simulink model "BMS_System"  (R2024a)
settings: Solver=VariableStepAuto  StartTime=0.0  StopTime=10.0  RelTol=1e-3
settings Model: DataDictionary=BMS_System_dict1.sldd  Creator=hirah  LastModifiedBy=hirah

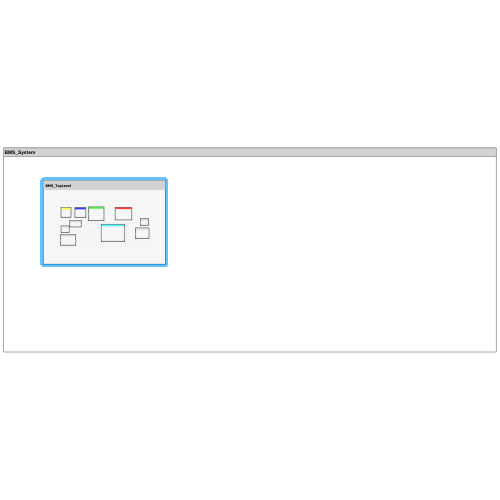
[thumbnail: Simulink's stored preview of the top-level diagram]
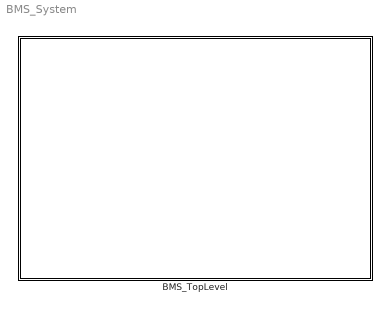
== system BMS_System ==
  BMS_TopLevel : Subsystem
      settings: PortSchema="{\"entries\":[{\"content\":{\"headerSize\":26,\"margin\":15,\"minimumSpacing\":25,\"sides\":[{\"content\":{},\"type\":\"ConnectorPlacement.EquallySpacedRectSide\",\"uuid\":\"0075fff4-e359-4ca3-82d3-62066e5371b3\"},{\"content\":{\"side\":\"RIGHT\"},\"type\":\"ConnectorPlacement.EquallySpacedRectSide\",\"uuid\":\"0762518f-8ff4-47a0-8585-614cecfccf10\"},{\"content\":{\"side\":\"TOP\"},\"type\":\"ConnectorPlacement.EquallySpacedRectSide\",\"uuid\":\"3af96ac8-a5e6-433b-be31-5dc09c2330cd\"}]},\"type\":\"ConnectorPlacement.EquallySpacedConnector\",\"uuid\":\"5c35ae06-51a0-47e4-81f3-25c096dd406a\"}],\"packageUris\":[\"http://schema.mathworks.com/mf0/Connector/R2020b\"],\"version\":\"1.0\"}"

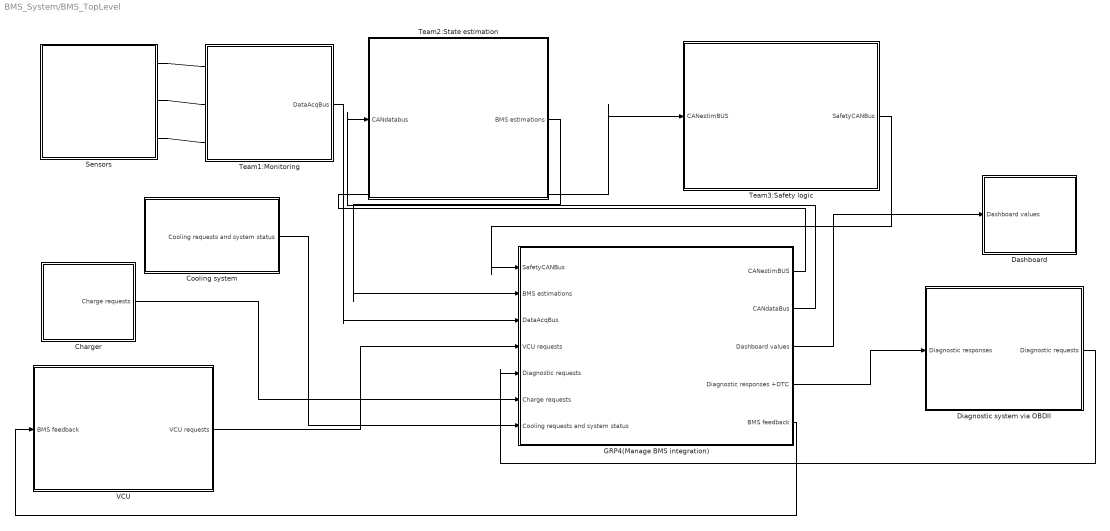
== system BMS_System/BMS_TopLevel ==
  Charger : Subsystem
      settings: PortSchema="{\"entries\":[{\"content\":{\"headerSize\":26,\"margin\":15,\"minimumSpacing\":25,\"sides\":[{\"content\":{},\"type\":\"ConnectorPlacement.EquallySpacedRectSide\",\"uuid\":\"cd2cdd02-8687-4a8c-9b6e-8ab5b03022cf\"},{\"content\":{\"connectorIds\":[\"Out1\"],\"side\":\"RIGHT\"},\"type\":\"ConnectorPlacement.EquallySpacedRectSide\",\"uuid\":\"c7d3337e-acaa-4958-9ee3-86e02c1b3b1e\"},{\"content\":{\"side\":\"TOP\"},\"type\":\"ConnectorPlacement.EquallySpacedRectSide\",\"uuid\":\"181ed1e6-99e4-4d5e-88b9-0d6c177ff349\"}]},\"type\":\"ConnectorPlacement.EquallySpacedConnector\",\"uuid\":\"35383a89-4be3-49fe-8681-3a2efe2b709c\"}],\"packageUris\":[\"http://schema.mathworks.com/mf0/Connector/R2020b\"],\"version\":\"1.0\"}"
  Cooling system : Subsystem
      settings: PortSchema="{\"entries\":[{\"content\":{\"headerSize\":26,\"margin\":15,\"minimumSpacing\":25,\"sides\":[{\"content\":{},\"type\":\"ConnectorPlacement.EquallySpacedRectSide\",\"uuid\":\"cd2cdd02-8687-4a8c-9b6e-8ab5b03022cf\"},{\"content\":{\"connectorIds\":[\"Out1\"],\"side\":\"RIGHT\"},\"type\":\"ConnectorPlacement.EquallySpacedRectSide\",\"uuid\":\"c7d3337e-acaa-4958-9ee3-86e02c1b3b1e\"},{\"content\":{\"side\":\"TOP\"},\"type\":\"ConnectorPlacement.EquallySpacedRectSide\",\"uuid\":\"181ed1e6-99e4-4d5e-88b9-0d6c177ff349\"}]},\"type\":\"ConnectorPlacement.EquallySpacedConnector\",\"uuid\":\"35383a89-4be3-49fe-8681-3a2efe2b709c\"}],\"packageUris\":[\"http://schema.mathworks.com/mf0/Connector/R2020b\"],\"version\":\"1.0\"}"
  Dashboard : Subsystem
      settings: PortSchema="{\"entries\":[{\"content\":{\"headerSize\":26,\"margin\":15,\"minimumSpacing\":25,\"sides\":[{\"content\":{\"connectorIds\":[\"In1\"]},\"type\":\"ConnectorPlacement.EquallySpacedRectSide\",\"uuid\":\"cd2cdd02-8687-4a8c-9b6e-8ab5b03022cf\"},{\"content\":{\"side\":\"RIGHT\"},\"type\":\"ConnectorPlacement.EquallySpacedRectSide\",\"uuid\":\"c7d3337e-acaa-4958-9ee3-86e02c1b3b1e\"},{\"content\":{\"side\":\"TOP\"},\"type\":\"ConnectorPlacement.EquallySpacedRectSide\",\"uuid\":\"181ed1e6-99e4-4d5e-88b9-0d6c177ff349\"}]},\"type\":\"ConnectorPlacement.EquallySpacedConnector\",\"uuid\":\"35383a89-4be3-49fe-8681-3a2efe2b709c\"}],\"packageUris\":[\"http://schema.mathworks.com/mf0/Connector/R2020b\"],\"version\":\"1.0\"}"
  Diagnostic system via OBDII : Subsystem
      settings: PortSchema="{\"entries\":[{\"content\":{\"headerSize\":26,\"margin\":15,\"minimumSpacing\":25,\"sides\":[{\"content\":{\"connectorIds\":[\"In1\"]},\"type\":\"ConnectorPlacement.EquallySpacedRectSide\",\"uuid\":\"cd2cdd02-8687-4a8c-9b6e-8ab5b03022cf\"},{\"content\":{\"connectorIds\":[\"Out1\"],\"side\":\"RIGHT\"},\"type\":\"ConnectorPlacement.EquallySpacedRectSide\",\"uuid\":\"c7d3337e-acaa-4958-9ee3-86e02c1b3b1e\"},{\"content\":{\"side\":\"TOP\"},\"type\":\"ConnectorPlacement.EquallySpacedRectSide\",\"uuid\":\"181ed1e6-99e4-4d5e-88b9-0d6c177ff349\"}]},\"type\":\"ConnectorPlacement.EquallySpacedConnector\",\"uuid\":\"35383a89-4be3-49fe-8681-3a2efe2b709c\"}],\"packageUris\":[\"http://schema.mathworks.com/mf0/Connector/R2020b\"],\"version\":\"1.0\"}"
  GRP4(Manage BMS integration) : Subsystem
      settings: PortSchema="{\"entries\":[{\"content\":{\"headerSize\":26,\"margin\":15,\"minimumSpacing\":25,\"sides\":[{\"content\":{\"connectorIds\":[\"In1\",\"In6\",\"In2\",\"In7\",\"In3\",\"In4\",\"In5\"]},\"type\":\"ConnectorPlacement.EquallySpacedRectSide\",\"uuid\":\"faff89d9-e9e4-4b6f-9f42-f9315910e0de\"},{\"content\":{\"connectorIds\":[\"Out1\",\"Out2\",\"Out3\",\"Out4\",\"Out5\"],\"side\":\"RIGHT\"},\"type\":\"ConnectorPlacement.EquallySpacedRectSide\",\"uuid\":\"9773bad6-87c4-4101-99c1-1d204d4e17cb\"},{\"content\":{\"side\":\"TOP\"},\"type\":\"ConnectorPlacement.EquallySpacedRectSide\",\"uuid\":\"573ffa45-035d-496a-acbc-febfae678741\"}]},\"type\":\"ConnectorPlacement.EquallySpacedConnector\",\"uuid\":\"e66d261f-d4c2-4899-bd49-de4415fbe12f\"}],\"packageUris\":[\"http://schema.mathworks.com/mf0/Connector/R2020b\"],\"version\":\"1.0\"}"
  Sensors : Subsystem
      settings: PortSchema="{\"entries\":[{\"content\":{\"headerSize\":26,\"margin\":15,\"minimumSpacing\":25,\"sides\":[{\"content\":{},\"type\":\"ConnectorPlacement.EquallySpacedRectSide\",\"uuid\":\"faff89d9-e9e4-4b6f-9f42-f9315910e0de\"},{\"content\":{\"connectorIds\":[\"RConn1\",\"RConn2\",\"RConn3\"],\"side\":\"RIGHT\"},\"type\":\"ConnectorPlacement.EquallySpacedRectSide\",\"uuid\":\"9773bad6-87c4-4101-99c1-1d204d4e17cb\"},{\"content\":{\"side\":\"TOP\"},\"type\":\"ConnectorPlacement.EquallySpacedRectSide\",\"uuid\":\"573ffa45-035d-496a-acbc-febfae678741\"}]},\"type\":\"ConnectorPlacement.EquallySpacedConnector\",\"uuid\":\"e66d261f-d4c2-4899-bd49-de4415fbe12f\"}],\"packageUris\":[\"http://schema.mathworks.com/mf0/Connector/R2020b\"],\"version\":\"1.0\"}"
  Team1:Monitoring : Subsystem
      settings: PortSchema="{\"entries\":[{\"content\":{\"headerSize\":26,\"margin\":15,\"minimumSpacing\":25,\"sides\":[{\"content\":{\"connectorIds\":[\"LConn1\",\"LConn2\",\"LConn3\"]},\"type\":\"ConnectorPlacement.EquallySpacedRectSide\",\"uuid\":\"cd2cdd02-8687-4a8c-9b6e-8ab5b03022cf\"},{\"content\":{\"connectorIds\":[\"Out1\"],\"side\":\"RIGHT\"},\"type\":\"ConnectorPlacement.EquallySpacedRectSide\",\"uuid\":\"c7d3337e-acaa-4958-9ee3-86e02c1b3b1e\"},{\"content\":{\"side\":\"TOP\"},\"type\":\"ConnectorPlacement.EquallySpacedRectSide\",\"uuid\":\"181ed1e6-99e4-4d5e-88b9-0d6c177ff349\"}]},\"type\":\"ConnectorPlacement.EquallySpacedConnector\",\"uuid\":\"35383a89-4be3-49fe-8681-3a2efe2b709c\"}],\"packageUris\":[\"http://schema.mathworks.com/mf0/Connector/R2020b\"],\"version\":\"1.0\"}"
  Team2:State estimation : Subsystem
      settings: PortSchema="{\"entries\":[{\"content\":{\"headerSize\":26,\"margin\":15,\"minimumSpacing\":25,\"sides\":[{\"content\":{\"connectorIds\":[\"In1\"]},\"type\":\"ConnectorPlacement.EquallySpacedRectSide\",\"uuid\":\"faff89d9-e9e4-4b6f-9f42-f9315910e0de\"},{\"content\":{\"connectorIds\":[\"Out1\"],\"side\":\"RIGHT\"},\"type\":\"ConnectorPlacement.EquallySpacedRectSide\",\"uuid\":\"9773bad6-87c4-4101-99c1-1d204d4e17cb\"},{\"content\":{\"side\":\"TOP\"},\"type\":\"ConnectorPlacement.EquallySpacedRectSide\",\"uuid\":\"573ffa45-035d-496a-acbc-febfae678741\"}]},\"type\":\"ConnectorPlacement.EquallySpacedConnector\",\"uuid\":\"e66d261f-d4c2-4899-bd49-de4415fbe12f\"}],\"packageUris\":[\"http://schema.mathworks.com/mf0/Connector/R2020b\"],\"version\":\"1.0\"}"
  Team3:Safety logic : Subsystem
      settings: PortSchema="{\"entries\":[{\"content\":{\"headerSize\":26,\"margin\":15,\"minimumSpacing\":25,\"sides\":[{\"content\":{\"connectorIds\":[\"In1\"]},\"type\":\"ConnectorPlacement.EquallySpacedRectSide\",\"uuid\":\"cd2cdd02-8687-4a8c-9b6e-8ab5b03022cf\"},{\"content\":{\"connectorIds\":[\"Out1\"],\"side\":\"RIGHT\"},\"type\":\"ConnectorPlacement.EquallySpacedRectSide\",\"uuid\":\"c7d3337e-acaa-4958-9ee3-86e02c1b3b1e\"},{\"content\":{\"side\":\"TOP\"},\"type\":\"ConnectorPlacement.EquallySpacedRectSide\",\"uuid\":\"181ed1e6-99e4-4d5e-88b9-0d6c177ff349\"}]},\"type\":\"ConnectorPlacement.EquallySpacedConnector\",\"uuid\":\"35383a89-4be3-49fe-8681-3a2efe2b709c\"}],\"packageUris\":[\"http://schema.mathworks.com/mf0/Connector/R2020b\"],\"version\":\"1.0\"}"
  VCU : Subsystem
      settings: PortSchema="{\"entries\":[{\"content\":{\"headerSize\":26,\"margin\":15,\"minimumSpacing\":25,\"sides\":[{\"content\":{\"connectorIds\":[\"In1\"]},\"type\":\"ConnectorPlacement.EquallySpacedRectSide\",\"uuid\":\"cd2cdd02-8687-4a8c-9b6e-8ab5b03022cf\"},{\"content\":{\"connectorIds\":[\"Out1\"],\"side\":\"RIGHT\"},\"type\":\"ConnectorPlacement.EquallySpacedRectSide\",\"uuid\":\"c7d3337e-acaa-4958-9ee3-86e02c1b3b1e\"},{\"content\":{\"side\":\"TOP\"},\"type\":\"ConnectorPlacement.EquallySpacedRectSide\",\"uuid\":\"181ed1e6-99e4-4d5e-88b9-0d6c177ff349\"}]},\"type\":\"ConnectorPlacement.EquallySpacedConnector\",\"uuid\":\"35383a89-4be3-49fe-8681-3a2efe2b709c\"}],\"packageUris\":[\"http://schema.mathworks.com/mf0/Connector/R2020b\"],\"version\":\"1.0\"}"
  wires:
  Team2:State estimation/1(BMS estimations) -> GRP4(Manage BMS integration)/6(BMS estimations)
  VCU/1(VCU requests) -> GRP4(Manage BMS integration)/7(VCU requests)
  GRP4(Manage BMS integration)/1(CANestimBUS) -> Team3:Safety logic/1(CANestimBUS)
  Team3:Safety logic/1(SafetyCANBus) -> GRP4(Manage BMS integration)/1(SafetyCANBus)
  GRP4(Manage BMS integration)/5(BMS feedback) -> VCU/1(BMS feedback)
  GRP4(Manage BMS integration)/4(Diagnostic responses +DTC) -> Diagnostic system via OBDII/1(Diagnostic responses)
  Diagnostic system via OBDII/1(Diagnostic requests) -> GRP4(Manage BMS integration)/3(Diagnostic requests)
  GRP4(Manage BMS integration)/3(Dashboard values) -> Dashboard/1(Dashboard values)
  Charger/1(Charge requests) -> GRP4(Manage BMS integration)/4(Charge requests)
  Cooling system/1(Cooling requests and system status) -> GRP4(Manage BMS integration)/5(Cooling requests and system status)
  Team1:Monitoring/1(DataAcqBus) -> GRP4(Manage BMS integration)/2(DataAcqBus)
  GRP4(Manage BMS integration)/2(CANdataBus) -> Team2:State estimation/1(CANdatabus)
  connections:
  Sensors/RConn2 -- Team1:Monitoring/LConn2
  Sensors/RConn1 -- Team1:Monitoring/LConn1
  Sensors/RConn3 -- Team1:Monitoring/LConn3

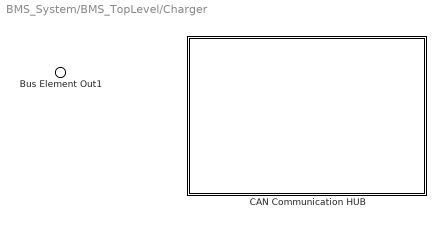
== system BMS_System/BMS_TopLevel/Charger ==
  CAN Communication HUB : Subsystem
      settings: PortSchema="{\"entries\":[{\"content\":{\"headerSize\":26,\"margin\":15,\"minimumSpacing\":25,\"sides\":[{\"content\":{},\"type\":\"ConnectorPlacement.EquallySpacedRectSide\",\"uuid\":\"5bf11642-2165-495a-8f16-07288b1b2a7f\"},{\"content\":{\"side\":\"RIGHT\"},\"type\":\"ConnectorPlacement.EquallySpacedRectSide\",\"uuid\":\"16013c05-30c7-4811-aab5-6705354ddbd6\"},{\"content\":{\"side\":\"TOP\"},\"type\":\"ConnectorPlacement.EquallySpacedRectSide\",\"uuid\":\"95109c83-3f97-4257-a072-0eae8b681641\"}]},\"type\":\"ConnectorPlacement.EquallySpacedConnector\",\"uuid\":\"ab507b5d-7f02-463f-8b22-b752f4ca7c99\"}],\"packageUris\":[\"http://schema.mathworks.com/mf0/Connector/R2020b\"],\"version\":\"1.0\"}"
  Bus Element Out1 : Outport  PortName=Charge requests

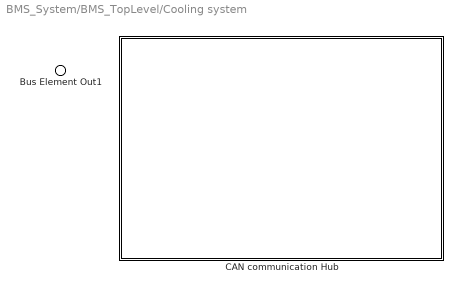
== system BMS_System/BMS_TopLevel/Cooling system ==
  CAN communication Hub : Subsystem
      settings: PortSchema="{\"entries\":[{\"content\":{\"headerSize\":26,\"margin\":15,\"minimumSpacing\":25,\"sides\":[{\"content\":{},\"type\":\"ConnectorPlacement.EquallySpacedRectSide\",\"uuid\":\"5bf11642-2165-495a-8f16-07288b1b2a7f\"},{\"content\":{\"side\":\"RIGHT\"},\"type\":\"ConnectorPlacement.EquallySpacedRectSide\",\"uuid\":\"16013c05-30c7-4811-aab5-6705354ddbd6\"},{\"content\":{\"side\":\"TOP\"},\"type\":\"ConnectorPlacement.EquallySpacedRectSide\",\"uuid\":\"95109c83-3f97-4257-a072-0eae8b681641\"}]},\"type\":\"ConnectorPlacement.EquallySpacedConnector\",\"uuid\":\"ab507b5d-7f02-463f-8b22-b752f4ca7c99\"}],\"packageUris\":[\"http://schema.mathworks.com/mf0/Connector/R2020b\"],\"version\":\"1.0\"}"
  Bus Element Out1 : Outport  PortName=Cooling requests and system status

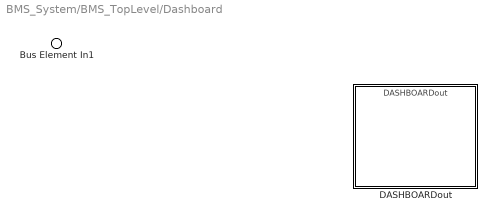
== system BMS_System/BMS_TopLevel/Dashboard ==
  Bus Element In1 : Inport  PortName=Dashboard values
  DASHBOARDout : ModelReference  ModelNameDialog=DASHBOARDout  SimulationMode=Normal  ModelReferenceVersion=1.2
      settings: PortSchema="{\"entries\":[{\"content\":{\"headerSize\":38,\"margin\":15,\"minimumSpacing\":25,\"sides\":[{\"content\":{},\"type\":\"ConnectorPlacement.EquallySpacedRectSide\",\"uuid\":\"442a0f05-4206-4dc5-b8c0-ef4408890997\"},{\"content\":{\"side\":\"RIGHT\"},\"type\":\"ConnectorPlacement.EquallySpacedRectSide\",\"uuid\":\"a731e2a3-c09d-4f46-98a5-6423e1f8e87d\"},{\"content\":{\"side\":\"TOP\"},\"type\":\"ConnectorPlacement.EquallySpacedRectSide\",\"uuid\":\"cd806d94-91fe-481e-8656-b1a7cedeabf9\"}]},\"type\":\"ConnectorPlacement.EquallySpacedConnector\",\"uuid\":\"cf8413cb-3c81-4bbe-84a6-0d7f87f95c7c\"}],\"packageUris\":[\"http://schema.mathworks.com/mf0/Connector/R2020b\"],\"version\":\"1.0\"}"

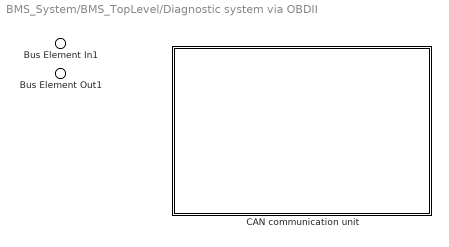
== system BMS_System/BMS_TopLevel/Diagnostic system via OBDII ==
  Bus Element In1 : Inport  PortName=Diagnostic responses
  CAN communication unit : Subsystem
      settings: PortSchema="{\"entries\":[{\"content\":{\"headerSize\":26,\"margin\":15,\"minimumSpacing\":25,\"sides\":[{\"content\":{},\"type\":\"ConnectorPlacement.EquallySpacedRectSide\",\"uuid\":\"442a0f05-4206-4dc5-b8c0-ef4408890997\"},{\"content\":{\"side\":\"RIGHT\"},\"type\":\"ConnectorPlacement.EquallySpacedRectSide\",\"uuid\":\"a731e2a3-c09d-4f46-98a5-6423e1f8e87d\"},{\"content\":{\"side\":\"TOP\"},\"type\":\"ConnectorPlacement.EquallySpacedRectSide\",\"uuid\":\"cd806d94-91fe-481e-8656-b1a7cedeabf9\"}]},\"type\":\"ConnectorPlacement.EquallySpacedConnector\",\"uuid\":\"cf8413cb-3c81-4bbe-84a6-0d7f87f95c7c\"}],\"packageUris\":[\"http://schema.mathworks.com/mf0/Connector/R2020b\"],\"version\":\"1.0\"}"
  Bus Element Out1 : Outport  PortName=Diagnostic requests

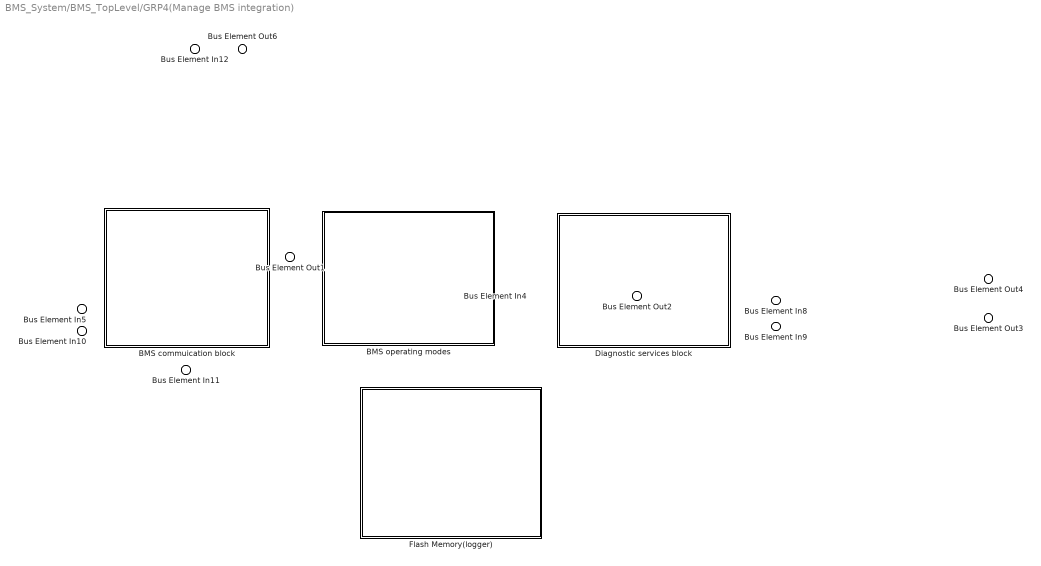
== system BMS_System/BMS_TopLevel/GRP4(Manage BMS integration) ==
  Bus Element In8 : Inport  PortName=SafetyCANBus
  Bus Element In12 : Inport  Port=2  PortName=DataAcqBus
  Bus Element In9 : Inport  Port=3  PortName=Diagnostic requests
  Bus Element In10 : Inport  Port=4  PortName=Charge requests
  Bus Element In11 : Inport  Port=5  PortName=Cooling requests and system status
  Bus Element In4 : Inport  Port=6  PortName=BMS estimations
  Bus Element In5 : Inport  Port=7  PortName=VCU requests
  BMS commuication block : Subsystem
      settings: PortSchema="{\"entries\":[{\"content\":{\"headerSize\":26,\"margin\":15,\"minimumSpacing\":25,\"sides\":[{\"content\":{},\"type\":\"ConnectorPlacement.EquallySpacedRectSide\",\"uuid\":\"04ec415f-b4bd-4017-972b-9e85e691a4fa\"},{\"content\":{\"side\":\"RIGHT\"},\"type\":\"ConnectorPlacement.EquallySpacedRectSide\",\"uuid\":\"35151384-2339-42ef-bb6e-a180feceabd8\"},{\"content\":{\"side\":\"TOP\"},\"type\":\"ConnectorPlacement.EquallySpacedRectSide\",\"uuid\":\"c25567f8-acdc-4fac-aea5-0e07a58d33ff\"},{\"content\":{\"side\":\"BOTTOM\"},\"type\":\"ConnectorPlacement.EquallySpacedRectSide\",\"uuid\":\"03d92b78-152a-4a99-a80a-d3186856140b\"}]},\"type\":\"ConnectorPlacement.EquallySpacedConnector\",\"uuid\":\"6bdc95ed-225b-47c7-9236-872fc0620aae\"}],\"packageUris\":[\"http://schema.mathworks.com/mf0/Connector/R2020b\"],\"version\":\"1.0\"}"
  BMS operating modes : Subsystem
      settings: PortSchema="{\"entries\":[{\"content\":{\"headerSize\":26,\"margin\":15,\"minimumSpacing\":25,\"sides\":[{\"content\":{},\"type\":\"ConnectorPlacement.EquallySpacedRectSide\",\"uuid\":\"faff89d9-e9e4-4b6f-9f42-f9315910e0de\"},{\"content\":{\"side\":\"RIGHT\"},\"type\":\"ConnectorPlacement.EquallySpacedRectSide\",\"uuid\":\"9773bad6-87c4-4101-99c1-1d204d4e17cb\"},{\"content\":{\"side\":\"TOP\"},\"type\":\"ConnectorPlacement.EquallySpacedRectSide\",\"uuid\":\"573ffa45-035d-496a-acbc-febfae678741\"}]},\"type\":\"ConnectorPlacement.EquallySpacedConnector\",\"uuid\":\"e66d261f-d4c2-4899-bd49-de4415fbe12f\"}],\"packageUris\":[\"http://schema.mathworks.com/mf0/Connector/R2020b\"],\"version\":\"1.0\"}"
  Diagnostic services block : Subsystem
      settings: PortSchema="{\"entries\":[{\"content\":{\"headerSize\":26,\"margin\":15,\"minimumSpacing\":25,\"sides\":[{\"content\":{},\"type\":\"ConnectorPlacement.EquallySpacedRectSide\",\"uuid\":\"04ec415f-b4bd-4017-972b-9e85e691a4fa\"},{\"content\":{\"side\":\"RIGHT\"},\"type\":\"ConnectorPlacement.EquallySpacedRectSide\",\"uuid\":\"35151384-2339-42ef-bb6e-a180feceabd8\"},{\"content\":{\"side\":\"TOP\"},\"type\":\"ConnectorPlacement.EquallySpacedRectSide\",\"uuid\":\"c25567f8-acdc-4fac-aea5-0e07a58d33ff\"}]},\"type\":\"ConnectorPlacement.EquallySpacedConnector\",\"uuid\":\"6bdc95ed-225b-47c7-9236-872fc0620aae\"}],\"packageUris\":[\"http://schema.mathworks.com/mf0/Connector/R2020b\"],\"version\":\"1.0\"}"
  Flash Memory(logger) : Subsystem
      settings: PortSchema="{\"entries\":[{\"content\":{\"headerSize\":26,\"margin\":15,\"minimumSpacing\":25,\"sides\":[{\"content\":{},\"type\":\"ConnectorPlacement.EquallySpacedRectSide\",\"uuid\":\"442a0f05-4206-4dc5-b8c0-ef4408890997\"},{\"content\":{\"side\":\"RIGHT\"},\"type\":\"ConnectorPlacement.EquallySpacedRectSide\",\"uuid\":\"a731e2a3-c09d-4f46-98a5-6423e1f8e87d\"},{\"content\":{\"side\":\"TOP\"},\"type\":\"ConnectorPlacement.EquallySpacedRectSide\",\"uuid\":\"cd806d94-91fe-481e-8656-b1a7cedeabf9\"}]},\"type\":\"ConnectorPlacement.EquallySpacedConnector\",\"uuid\":\"cf8413cb-3c81-4bbe-84a6-0d7f87f95c7c\"}],\"packageUris\":[\"http://schema.mathworks.com/mf0/Connector/R2020b\"],\"version\":\"1.0\"}"
  Bus Element Out1 : Outport  PortName=CANestimBUS
  Bus Element Out6 : Outport  Port=2  PortName=CANdataBus
  Bus Element Out4 : Outport  Port=3  PortName=Dashboard values
  Bus Element Out3 : Outport  Port=4  PortName=Diagnostic responses +DTC
  Bus Element Out2 : Outport  Port=5  PortName=BMS feedback

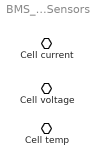
== system BMS_System/BMS_TopLevel/Sensors ==
  Cell current : PMIOPort  Side=Right
  Cell voltage : PMIOPort  Port=2  Side=Right
  Cell temp : PMIOPort  Port=3  Side=Right

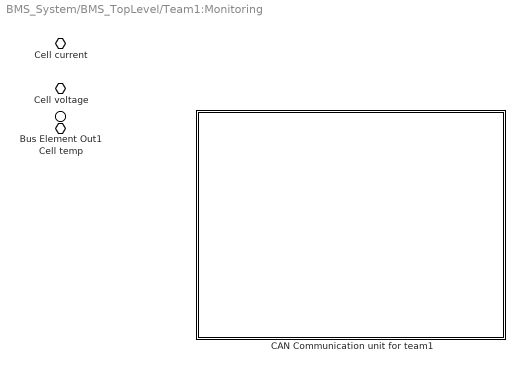
== system BMS_System/BMS_TopLevel/Team1:Monitoring ==
  CAN Communication unit for team1 : Subsystem
      settings: PortSchema="{\"entries\":[{\"content\":{\"headerSize\":26,\"margin\":15,\"minimumSpacing\":25,\"sides\":[{\"content\":{},\"type\":\"ConnectorPlacement.EquallySpacedRectSide\",\"uuid\":\"5bf11642-2165-495a-8f16-07288b1b2a7f\"},{\"content\":{\"side\":\"RIGHT\"},\"type\":\"ConnectorPlacement.EquallySpacedRectSide\",\"uuid\":\"16013c05-30c7-4811-aab5-6705354ddbd6\"},{\"content\":{\"side\":\"TOP\"},\"type\":\"ConnectorPlacement.EquallySpacedRectSide\",\"uuid\":\"95109c83-3f97-4257-a072-0eae8b681641\"}]},\"type\":\"ConnectorPlacement.EquallySpacedConnector\",\"uuid\":\"ab507b5d-7f02-463f-8b22-b752f4ca7c99\"}],\"packageUris\":[\"http://schema.mathworks.com/mf0/Connector/R2020b\"],\"version\":\"1.0\"}"
  Cell current : PMIOPort  Side=Left  ConnectionType=Connection: foundation.electrical.eight_phase
  Cell voltage : PMIOPort  Port=2  Side=Left
  Cell temp : PMIOPort  Port=3  Side=Left
  Bus Element Out1 : Outport  PortName=DataAcqBus

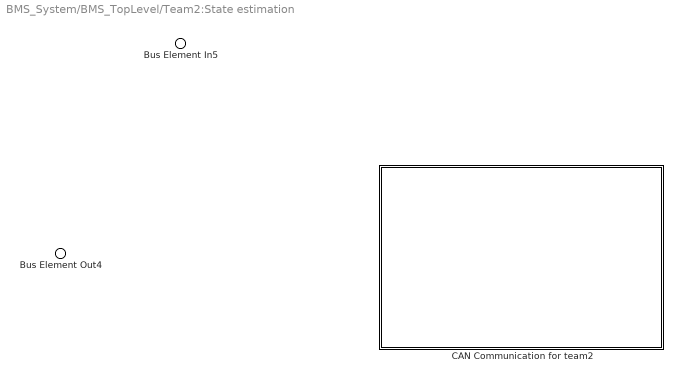
== system BMS_System/BMS_TopLevel/Team2:State estimation ==
  Bus Element In5 : Inport  PortName=CANdatabus
  CAN Communication for team2 : Subsystem
      settings: PortSchema="{\"entries\":[{\"content\":{\"headerSize\":26,\"margin\":15,\"minimumSpacing\":25,\"sides\":[{\"content\":{},\"type\":\"ConnectorPlacement.EquallySpacedRectSide\",\"uuid\":\"5bf11642-2165-495a-8f16-07288b1b2a7f\"},{\"content\":{\"side\":\"RIGHT\"},\"type\":\"ConnectorPlacement.EquallySpacedRectSide\",\"uuid\":\"16013c05-30c7-4811-aab5-6705354ddbd6\"},{\"content\":{\"side\":\"TOP\"},\"type\":\"ConnectorPlacement.EquallySpacedRectSide\",\"uuid\":\"95109c83-3f97-4257-a072-0eae8b681641\"}]},\"type\":\"ConnectorPlacement.EquallySpacedConnector\",\"uuid\":\"ab507b5d-7f02-463f-8b22-b752f4ca7c99\"}],\"packageUris\":[\"http://schema.mathworks.com/mf0/Connector/R2020b\"],\"version\":\"1.0\"}"
  Bus Element Out4 : Outport  PortName=BMS estimations

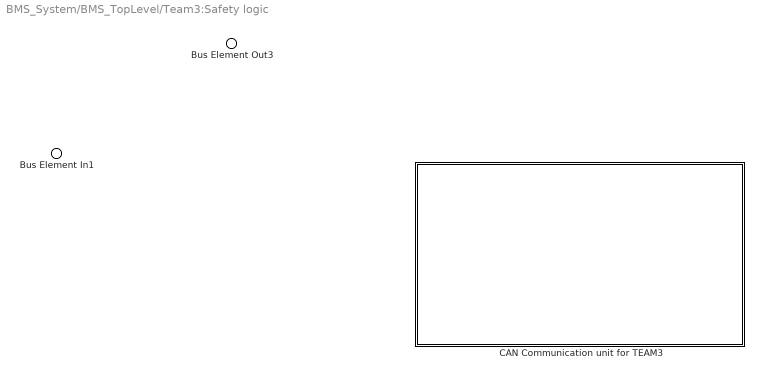
== system BMS_System/BMS_TopLevel/Team3:Safety logic ==
  Bus Element In1 : Inport  PortName=CANestimBUS
  CAN Communication unit for TEAM3 : Subsystem
      settings: PortSchema="{\"entries\":[{\"content\":{\"headerSize\":26,\"margin\":15,\"minimumSpacing\":25,\"sides\":[{\"content\":{},\"type\":\"ConnectorPlacement.EquallySpacedRectSide\",\"uuid\":\"5bf11642-2165-495a-8f16-07288b1b2a7f\"},{\"content\":{\"side\":\"RIGHT\"},\"type\":\"ConnectorPlacement.EquallySpacedRectSide\",\"uuid\":\"16013c05-30c7-4811-aab5-6705354ddbd6\"},{\"content\":{\"side\":\"TOP\"},\"type\":\"ConnectorPlacement.EquallySpacedRectSide\",\"uuid\":\"95109c83-3f97-4257-a072-0eae8b681641\"}]},\"type\":\"ConnectorPlacement.EquallySpacedConnector\",\"uuid\":\"ab507b5d-7f02-463f-8b22-b752f4ca7c99\"}],\"packageUris\":[\"http://schema.mathworks.com/mf0/Connector/R2020b\"],\"version\":\"1.0\"}"
  Bus Element Out3 : Outport  PortName=SafetyCANBus

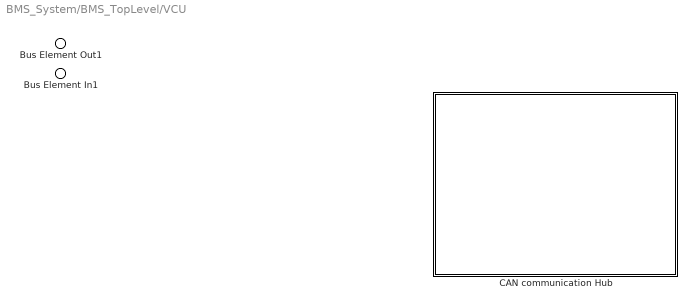
== system BMS_System/BMS_TopLevel/VCU ==
  Bus Element In1 : Inport  PortName=BMS feedback
  CAN communication Hub : Subsystem
      settings: PortSchema="{\"entries\":[{\"content\":{\"headerSize\":26,\"margin\":15,\"minimumSpacing\":25,\"sides\":[{\"content\":{},\"type\":\"ConnectorPlacement.EquallySpacedRectSide\",\"uuid\":\"442a0f05-4206-4dc5-b8c0-ef4408890997\"},{\"content\":{\"side\":\"RIGHT\"},\"type\":\"ConnectorPlacement.EquallySpacedRectSide\",\"uuid\":\"a731e2a3-c09d-4f46-98a5-6423e1f8e87d\"},{\"content\":{\"side\":\"TOP\"},\"type\":\"ConnectorPlacement.EquallySpacedRectSide\",\"uuid\":\"cd806d94-91fe-481e-8656-b1a7cedeabf9\"}]},\"type\":\"ConnectorPlacement.EquallySpacedConnector\",\"uuid\":\"cf8413cb-3c81-4bbe-84a6-0d7f87f95c7c\"}],\"packageUris\":[\"http://schema.mathworks.com/mf0/Connector/R2020b\"],\"version\":\"1.0\"}"
  Bus Element Out1 : Outport  PortName=VCU requests

== system BMS_System/BMS_TopLevel/Charger/CAN Communication HUB ==
  "CAN RX communication " : ModelReference  ModelNameDialog=Component_1  SimulationMode=Normal  ModelReferenceVersion=1.1
      settings: PortSchema="{\"entries\":[{\"content\":{\"headerSize\":38,\"margin\":15,\"minimumSpacing\":25,\"sides\":[{\"content\":{},\"type\":\"ConnectorPlacement.EquallySpacedRectSide\",\"uuid\":\"5bf11642-2165-495a-8f16-07288b1b2a7f\"},{\"content\":{\"side\":\"RIGHT\"},\"type\":\"ConnectorPlacement.EquallySpacedRectSide\",\"uuid\":\"16013c05-30c7-4811-aab5-6705354ddbd6\"},{\"content\":{\"side\":\"TOP\"},\"type\":\"ConnectorPlacement.EquallySpacedRectSide\",\"uuid\":\"95109c83-3f97-4257-a072-0eae8b681641\"}]},\"type\":\"ConnectorPlacement.EquallySpacedConnector\",\"uuid\":\"ab507b5d-7f02-463f-8b22-b752f4ca7c99\"}],\"packageUris\":[\"http://schema.mathworks.com/mf0/Connector/R2020b\"],\"version\":\"1.0\"}"
  CAN TX communication : ModelReference  ModelNameDialog=CANTXcommunication  SimulationMode=Normal  ModelReferenceVersion=1.1
      settings: PortSchema="{\"entries\":[{\"content\":{\"headerSize\":38,\"margin\":15,\"minimumSpacing\":25,\"sides\":[{\"content\":{},\"type\":\"ConnectorPlacement.EquallySpacedRectSide\",\"uuid\":\"5bf11642-2165-495a-8f16-07288b1b2a7f\"},{\"content\":{\"side\":\"RIGHT\"},\"type\":\"ConnectorPlacement.EquallySpacedRectSide\",\"uuid\":\"16013c05-30c7-4811-aab5-6705354ddbd6\"},{\"content\":{\"side\":\"TOP\"},\"type\":\"ConnectorPlacement.EquallySpacedRectSide\",\"uuid\":\"95109c83-3f97-4257-a072-0eae8b681641\"}]},\"type\":\"ConnectorPlacement.EquallySpacedConnector\",\"uuid\":\"ab507b5d-7f02-463f-8b22-b752f4ca7c99\"}],\"packageUris\":[\"http://schema.mathworks.com/mf0/Connector/R2020b\"],\"version\":\"1.0\"}"

== system BMS_System/BMS_TopLevel/Cooling system/CAN communication Hub ==
  CAN RX communication unit : ModelReference  ModelNameDialog=CANRXcommunicationunit_1  SimulationMode=Normal  ModelReferenceVersion=1.1
      settings: PortSchema="{\"entries\":[{\"content\":{\"headerSize\":38,\"margin\":15,\"minimumSpacing\":25,\"sides\":[{\"content\":{},\"type\":\"ConnectorPlacement.EquallySpacedRectSide\",\"uuid\":\"5bf11642-2165-495a-8f16-07288b1b2a7f\"},{\"content\":{\"side\":\"RIGHT\"},\"type\":\"ConnectorPlacement.EquallySpacedRectSide\",\"uuid\":\"16013c05-30c7-4811-aab5-6705354ddbd6\"},{\"content\":{\"side\":\"TOP\"},\"type\":\"ConnectorPlacement.EquallySpacedRectSide\",\"uuid\":\"95109c83-3f97-4257-a072-0eae8b681641\"}]},\"type\":\"ConnectorPlacement.EquallySpacedConnector\",\"uuid\":\"ab507b5d-7f02-463f-8b22-b752f4ca7c99\"}],\"packageUris\":[\"http://schema.mathworks.com/mf0/Connector/R2020b\"],\"version\":\"1.0\"}"
  CAN TX communication unit : ModelReference  ModelNameDialog=CANTXcommunicationunit_2  SimulationMode=Normal  ModelReferenceVersion=1.1
      settings: PortSchema="{\"entries\":[{\"content\":{\"headerSize\":38,\"margin\":15,\"minimumSpacing\":25,\"sides\":[{\"content\":{},\"type\":\"ConnectorPlacement.EquallySpacedRectSide\",\"uuid\":\"5bf11642-2165-495a-8f16-07288b1b2a7f\"},{\"content\":{\"side\":\"RIGHT\"},\"type\":\"ConnectorPlacement.EquallySpacedRectSide\",\"uuid\":\"16013c05-30c7-4811-aab5-6705354ddbd6\"},{\"content\":{\"side\":\"TOP\"},\"type\":\"ConnectorPlacement.EquallySpacedRectSide\",\"uuid\":\"95109c83-3f97-4257-a072-0eae8b681641\"}]},\"type\":\"ConnectorPlacement.EquallySpacedConnector\",\"uuid\":\"ab507b5d-7f02-463f-8b22-b752f4ca7c99\"}],\"packageUris\":[\"http://schema.mathworks.com/mf0/Connector/R2020b\"],\"version\":\"1.0\"}"

== system BMS_System/BMS_TopLevel/Diagnostic system via OBDII/CAN communication unit ==
  CAN RX communication : ModelReference  ModelNameDialog=CANRXcommunication  SimulationMode=Normal  ModelReferenceVersion=1.2
      settings: PortSchema="{\"entries\":[{\"content\":{\"headerSize\":38,\"margin\":15,\"minimumSpacing\":25,\"sides\":[{\"content\":{},\"type\":\"ConnectorPlacement.EquallySpacedRectSide\",\"uuid\":\"442a0f05-4206-4dc5-b8c0-ef4408890997\"},{\"content\":{\"side\":\"RIGHT\"},\"type\":\"ConnectorPlacement.EquallySpacedRectSide\",\"uuid\":\"a731e2a3-c09d-4f46-98a5-6423e1f8e87d\"},{\"content\":{\"side\":\"TOP\"},\"type\":\"ConnectorPlacement.EquallySpacedRectSide\",\"uuid\":\"cd806d94-91fe-481e-8656-b1a7cedeabf9\"}]},\"type\":\"ConnectorPlacement.EquallySpacedConnector\",\"uuid\":\"cf8413cb-3c81-4bbe-84a6-0d7f87f95c7c\"}],\"packageUris\":[\"http://schema.mathworks.com/mf0/Connector/R2020b\"],\"version\":\"1.0\"}"
  CAN TX communication : ModelReference  ModelNameDialog=CANTXcommunication_1  SimulationMode=Normal  ModelReferenceVersion=1.2
      settings: PortSchema="{\"entries\":[{\"content\":{\"headerSize\":38,\"margin\":15,\"minimumSpacing\":25,\"sides\":[{\"content\":{},\"type\":\"ConnectorPlacement.EquallySpacedRectSide\",\"uuid\":\"442a0f05-4206-4dc5-b8c0-ef4408890997\"},{\"content\":{\"side\":\"RIGHT\"},\"type\":\"ConnectorPlacement.EquallySpacedRectSide\",\"uuid\":\"a731e2a3-c09d-4f46-98a5-6423e1f8e87d\"},{\"content\":{\"side\":\"TOP\"},\"type\":\"ConnectorPlacement.EquallySpacedRectSide\",\"uuid\":\"cd806d94-91fe-481e-8656-b1a7cedeabf9\"}]},\"type\":\"ConnectorPlacement.EquallySpacedConnector\",\"uuid\":\"cf8413cb-3c81-4bbe-84a6-0d7f87f95c7c\"}],\"packageUris\":[\"http://schema.mathworks.com/mf0/Connector/R2020b\"],\"version\":\"1.0\"}"

== system BMS_System/BMS_TopLevel/GRP4(Manage BMS integration)/BMS commuication block ==

== system BMS_System/BMS_TopLevel/GRP4(Manage BMS integration)/BMS operating modes ==
  ModeManager : ModelReference  ModelNameDialog=ModeManager_1  SimulationMode=Normal  ModelReferenceVersion=1.10
      settings: PortSchema="{\"entries\":[{\"content\":{\"headerSize\":38,\"margin\":15,\"minimumSpacing\":25,\"sides\":[{\"content\":{},\"type\":\"ConnectorPlacement.EquallySpacedRectSide\",\"uuid\":\"442a0f05-4206-4dc5-b8c0-ef4408890997\"},{\"content\":{\"side\":\"RIGHT\"},\"type\":\"ConnectorPlacement.EquallySpacedRectSide\",\"uuid\":\"a731e2a3-c09d-4f46-98a5-6423e1f8e87d\"},{\"content\":{\"side\":\"TOP\"},\"type\":\"ConnectorPlacement.EquallySpacedRectSide\",\"uuid\":\"cd806d94-91fe-481e-8656-b1a7cedeabf9\"}]},\"type\":\"ConnectorPlacement.EquallySpacedConnector\",\"uuid\":\"cf8413cb-3c81-4bbe-84a6-0d7f87f95c7c\"}],\"packageUris\":[\"http://schema.mathworks.com/mf0/Connector/R2020b\"],\"version\":\"1.0\"}"

== system BMS_System/BMS_TopLevel/GRP4(Manage BMS integration)/Diagnostic services block ==
  UDS services : ModelReference  ModelNameDialog=UDSservices  SimulationMode=Normal  ModelReferenceVersion=1.2
      settings: PortSchema="{\"entries\":[{\"content\":{\"headerSize\":38,\"margin\":15,\"minimumSpacing\":25,\"sides\":[{\"content\":{},\"type\":\"ConnectorPlacement.EquallySpacedRectSide\",\"uuid\":\"442a0f05-4206-4dc5-b8c0-ef4408890997\"},{\"content\":{\"side\":\"RIGHT\"},\"type\":\"ConnectorPlacement.EquallySpacedRectSide\",\"uuid\":\"a731e2a3-c09d-4f46-98a5-6423e1f8e87d\"},{\"content\":{\"side\":\"TOP\"},\"type\":\"ConnectorPlacement.EquallySpacedRectSide\",\"uuid\":\"cd806d94-91fe-481e-8656-b1a7cedeabf9\"}]},\"type\":\"ConnectorPlacement.EquallySpacedConnector\",\"uuid\":\"cf8413cb-3c81-4bbe-84a6-0d7f87f95c7c\"}],\"packageUris\":[\"http://schema.mathworks.com/mf0/Connector/R2020b\"],\"version\":\"1.0\"}"

== system BMS_System/BMS_TopLevel/GRP4(Manage BMS integration)/Flash Memory(logger) ==
  LoggerFile : ModelReference  ModelNameDialog=LoggerFile  SimulationMode=Normal  ModelReferenceVersion=1.4
      settings: PortSchema="{\"entries\":[{\"content\":{\"headerSize\":38,\"margin\":15,\"minimumSpacing\":25,\"sides\":[{\"content\":{},\"type\":\"ConnectorPlacement.EquallySpacedRectSide\",\"uuid\":\"442a0f05-4206-4dc5-b8c0-ef4408890997\"},{\"content\":{\"side\":\"RIGHT\"},\"type\":\"ConnectorPlacement.EquallySpacedRectSide\",\"uuid\":\"a731e2a3-c09d-4f46-98a5-6423e1f8e87d\"},{\"content\":{\"side\":\"TOP\"},\"type\":\"ConnectorPlacement.EquallySpacedRectSide\",\"uuid\":\"cd806d94-91fe-481e-8656-b1a7cedeabf9\"}]},\"type\":\"ConnectorPlacement.EquallySpacedConnector\",\"uuid\":\"cf8413cb-3c81-4bbe-84a6-0d7f87f95c7c\"}],\"packageUris\":[\"http://schema.mathworks.com/mf0/Connector/R2020b\"],\"version\":\"1.0\"}"

== system BMS_System/BMS_TopLevel/Team1:Monitoring/CAN Communication unit for team1 ==
  CAN TX communication module : ModelReference  ModelNameDialog=CANcommunicationmodule  SimulationMode=Normal  ModelReferenceVersion=1.4
      settings: PortSchema="{\"entries\":[{\"content\":{\"headerSize\":38,\"margin\":15,\"minimumSpacing\":25,\"sides\":[{\"content\":{},\"type\":\"ConnectorPlacement.EquallySpacedRectSide\",\"uuid\":\"5bf11642-2165-495a-8f16-07288b1b2a7f\"},{\"content\":{\"side\":\"RIGHT\"},\"type\":\"ConnectorPlacement.EquallySpacedRectSide\",\"uuid\":\"16013c05-30c7-4811-aab5-6705354ddbd6\"},{\"content\":{\"side\":\"TOP\"},\"type\":\"ConnectorPlacement.EquallySpacedRectSide\",\"uuid\":\"95109c83-3f97-4257-a072-0eae8b681641\"}]},\"type\":\"ConnectorPlacement.EquallySpacedConnector\",\"uuid\":\"ab507b5d-7f02-463f-8b22-b752f4ca7c99\"}],\"packageUris\":[\"http://schema.mathworks.com/mf0/Connector/R2020b\"],\"version\":\"1.0\"}"

== system BMS_System/BMS_TopLevel/Team2:State estimation/CAN Communication for team2 ==
  CAN RX communication unit : ModelReference  ModelNameDialog=CANRXcommunicationunit  SimulationMode=Normal  ModelReferenceVersion=1.2
      settings: PortSchema="{\"entries\":[{\"content\":{\"headerSize\":38,\"margin\":15,\"minimumSpacing\":25,\"sides\":[{\"content\":{},\"type\":\"ConnectorPlacement.EquallySpacedRectSide\",\"uuid\":\"5bf11642-2165-495a-8f16-07288b1b2a7f\"},{\"content\":{\"side\":\"RIGHT\"},\"type\":\"ConnectorPlacement.EquallySpacedRectSide\",\"uuid\":\"16013c05-30c7-4811-aab5-6705354ddbd6\"},{\"content\":{\"side\":\"TOP\"},\"type\":\"ConnectorPlacement.EquallySpacedRectSide\",\"uuid\":\"95109c83-3f97-4257-a072-0eae8b681641\"}]},\"type\":\"ConnectorPlacement.EquallySpacedConnector\",\"uuid\":\"ab507b5d-7f02-463f-8b22-b752f4ca7c99\"}],\"packageUris\":[\"http://schema.mathworks.com/mf0/Connector/R2020b\"],\"version\":\"1.0\"}"
  CAN TX communication unit : ModelReference  ModelNameDialog=CANTXcommunicationunit  SimulationMode=Normal  ModelReferenceVersion=1.3
      settings: PortSchema="{\"entries\":[{\"content\":{\"headerSize\":38,\"margin\":15,\"minimumSpacing\":25,\"sides\":[{\"content\":{},\"type\":\"ConnectorPlacement.EquallySpacedRectSide\",\"uuid\":\"5bf11642-2165-495a-8f16-07288b1b2a7f\"},{\"content\":{\"side\":\"RIGHT\"},\"type\":\"ConnectorPlacement.EquallySpacedRectSide\",\"uuid\":\"16013c05-30c7-4811-aab5-6705354ddbd6\"},{\"content\":{\"side\":\"TOP\"},\"type\":\"ConnectorPlacement.EquallySpacedRectSide\",\"uuid\":\"95109c83-3f97-4257-a072-0eae8b681641\"}]},\"type\":\"ConnectorPlacement.EquallySpacedConnector\",\"uuid\":\"ab507b5d-7f02-463f-8b22-b752f4ca7c99\"}],\"packageUris\":[\"http://schema.mathworks.com/mf0/Connector/R2020b\"],\"version\":\"1.0\"}"

== system BMS_System/BMS_TopLevel/Team3:Safety logic/CAN Communication unit for TEAM3 ==
  CAN RX communication unit : ModelReference  ModelNameDialog=Component  SimulationMode=Normal  ModelReferenceVersion=1.1
      settings: PortSchema="{\"entries\":[{\"content\":{\"headerSize\":38,\"margin\":15,\"minimumSpacing\":25,\"sides\":[{\"content\":{},\"type\":\"ConnectorPlacement.EquallySpacedRectSide\",\"uuid\":\"5bf11642-2165-495a-8f16-07288b1b2a7f\"},{\"content\":{\"side\":\"RIGHT\"},\"type\":\"ConnectorPlacement.EquallySpacedRectSide\",\"uuid\":\"16013c05-30c7-4811-aab5-6705354ddbd6\"},{\"content\":{\"side\":\"TOP\"},\"type\":\"ConnectorPlacement.EquallySpacedRectSide\",\"uuid\":\"95109c83-3f97-4257-a072-0eae8b681641\"}]},\"type\":\"ConnectorPlacement.EquallySpacedConnector\",\"uuid\":\"ab507b5d-7f02-463f-8b22-b752f4ca7c99\"}],\"packageUris\":[\"http://schema.mathworks.com/mf0/Connector/R2020b\"],\"version\":\"1.0\"}"
  CAN TX communication unit : ModelReference  ModelNameDialog=CANTXcommunicationunit_1  SimulationMode=Normal  ModelReferenceVersion=1.1
      settings: PortSchema="{\"entries\":[{\"content\":{\"headerSize\":38,\"margin\":15,\"minimumSpacing\":25,\"sides\":[{\"content\":{},\"type\":\"ConnectorPlacement.EquallySpacedRectSide\",\"uuid\":\"5bf11642-2165-495a-8f16-07288b1b2a7f\"},{\"content\":{\"side\":\"RIGHT\"},\"type\":\"ConnectorPlacement.EquallySpacedRectSide\",\"uuid\":\"16013c05-30c7-4811-aab5-6705354ddbd6\"},{\"content\":{\"side\":\"TOP\"},\"type\":\"ConnectorPlacement.EquallySpacedRectSide\",\"uuid\":\"95109c83-3f97-4257-a072-0eae8b681641\"}]},\"type\":\"ConnectorPlacement.EquallySpacedConnector\",\"uuid\":\"ab507b5d-7f02-463f-8b22-b752f4ca7c99\"}],\"packageUris\":[\"http://schema.mathworks.com/mf0/Connector/R2020b\"],\"version\":\"1.0\"}"

== system BMS_System/BMS_TopLevel/VCU/CAN communication Hub ==
  CAN RX communication unit : ModelReference  ModelNameDialog=CANRXcommunicationunit_2  SimulationMode=Normal  ModelReferenceVersion=1.2
      settings: PortSchema="{\"entries\":[{\"content\":{\"headerSize\":38,\"margin\":15,\"minimumSpacing\":25,\"sides\":[{\"content\":{},\"type\":\"ConnectorPlacement.EquallySpacedRectSide\",\"uuid\":\"442a0f05-4206-4dc5-b8c0-ef4408890997\"},{\"content\":{\"side\":\"RIGHT\"},\"type\":\"ConnectorPlacement.EquallySpacedRectSide\",\"uuid\":\"a731e2a3-c09d-4f46-98a5-6423e1f8e87d\"},{\"content\":{\"side\":\"TOP\"},\"type\":\"ConnectorPlacement.EquallySpacedRectSide\",\"uuid\":\"cd806d94-91fe-481e-8656-b1a7cedeabf9\"}]},\"type\":\"ConnectorPlacement.EquallySpacedConnector\",\"uuid\":\"cf8413cb-3c81-4bbe-84a6-0d7f87f95c7c\"}],\"packageUris\":[\"http://schema.mathworks.com/mf0/Connector/R2020b\"],\"version\":\"1.0\"}"
  CAN TX communication unit : ModelReference  ModelNameDialog=CANTXcommunicationunit_4  SimulationMode=Normal  ModelReferenceVersion=1.3
      settings: PortSchema="{\"entries\":[{\"content\":{\"headerSize\":38,\"margin\":15,\"minimumSpacing\":25,\"sides\":[{\"content\":{},\"type\":\"ConnectorPlacement.EquallySpacedRectSide\",\"uuid\":\"442a0f05-4206-4dc5-b8c0-ef4408890997\"},{\"content\":{\"side\":\"RIGHT\"},\"type\":\"ConnectorPlacement.EquallySpacedRectSide\",\"uuid\":\"a731e2a3-c09d-4f46-98a5-6423e1f8e87d\"},{\"content\":{\"side\":\"TOP\"},\"type\":\"ConnectorPlacement.EquallySpacedRectSide\",\"uuid\":\"cd806d94-91fe-481e-8656-b1a7cedeabf9\"}]},\"type\":\"ConnectorPlacement.EquallySpacedConnector\",\"uuid\":\"cf8413cb-3c81-4bbe-84a6-0d7f87f95c7c\"}],\"packageUris\":[\"http://schema.mathworks.com/mf0/Connector/R2020b\"],\"version\":\"1.0\"}"
